simulink library "did"  (R2021b)
settings: Solver=VariableStepAuto  StartTime=0.0  StopTime=10.0  RelTol=1e-3
undefined symbols (not defined in the file or in its folder): ADID_DODRange_pct, ADID_SOCRange_pct, ADID_TempRange_C, DiscIntNeverNeededParam, ENUM_CHRGPLUGSTA_AC, ENUM_CHRGPLUGSTA_DC, ENUM_CHRGPLUGSTA_NONE, ENUM_DRIVETRAIN_AWD, ENUM_DRIVETRAIN_FWD, ENUM_DRIVETRAIN_RWD, ENUM_EXTCHRGSTS_CHARGING, ENUM_OBCV2LSTA_WORKING, ENUM_PWRSTASW_READY, ENUM_VEHICLETYPE_D31HAWD, ENUM_VEHICLETYPE_D31HRWD, HOUR2SEC, HUNDRED, KDID_CPSAVehSpdThres_kph, KDID_DIDModelVersion_raw, KDID_DoDChrgCycle_s, KDID_FiveKmEquivEnergy_Wh, KDID_FlashInitDIDModelVersion_raw, KDID_IPSAVehSpdThres_kph, KDID_PropActiveTripThres_s, KDID_PSARResetThres_sec, KDID_RESSCNTSDODRNGAXIS_enum, KDID_RESSTIMESOCRNGAXIS_enum, KDID_RESSTTEMPRNGAXIS_enum, KDID_WarnUpPropActiveThres_s, KDID_WarnUpVehOperIdleThres_mph, KDID_WarnUpVehOperIdleThres_s, KDID_WarnUpVehOperThres_mph, KDID_WarnUpVehOperThres_s, KPH2MPH, KXX2XX, MINUSONE_FLOAT, ONE_FLOAT, ONE_INT, ONE_INT16, ONE_PERCENT, TRUE, UINT16_MAX, UINT32_MAX, XX2KXX, ZERO_FLOAT, ZERO_INT, ZERO_INT16, ZERO_INT32
libraries: hcu_lib x112, simulink x10, nmm x1
(part 4 of 4)

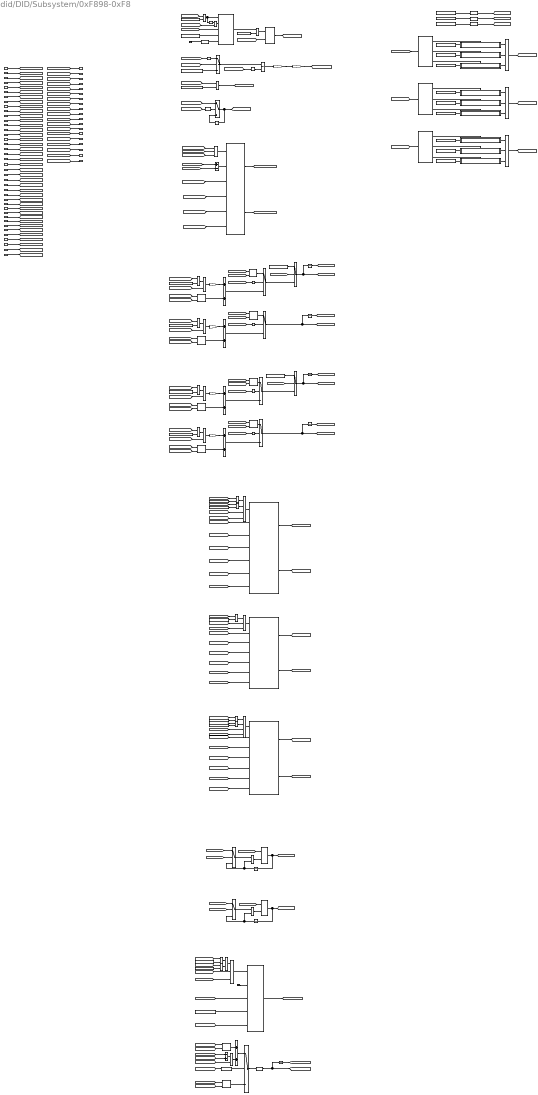
== system did/DID/Subsystem/0xF898-0xF8 ==
  note: 0xF89C: Electric Traction Motor A Total Output Energy
  note: 0xF898, 0xF899: Energy Storage System Depth of Discharge Counter
  note: 0xF89A: Energy Storage System Tracking Tables
  note: 0xF89D: Electric Traction Motor B Total Output Energy
  note: 0xF895: Average Battery Pack Temperature
  note: 0xF894: Minimum and Maximum Pack Temperature
  note: 0xF8A9-E: Energy Storage Accumulated Time at State of Charge
  VDID_HVBattPwr_kW : Inport
  task_time_s : Inport  Port=2
  VINP_CANMsgValidBMS1_flg : Inport  Port=3
  VDID_NoteAResetCondition_flg : Inport  Port=4
  VINP_FlashRESSCNTDODRNGR_cnt : Inport  Port=5
  VINP_FlashRESSCNTDODRNGL_cnt : Inport  Port=6
  VINP_RrMCUDCBusCurr_A : Inport  Port=7
  VINP_RrMCUDCBusVolt_V : Inport  Port=8
  VINP_FlashETMATOER_kWh : Inport  Port=9
  VINP_FlashETMATOEL_kWh : Inport  Port=10
  VINP_CANMsgValidMCUBR1_flg : Inport  Port=11
  VINP_FrMCUDCBusCurr_A : Inport  Port=12
  VINP_FrMCUDCBusVolt_V : Inport  Port=13
  VINP_FlashETMBTOER_kWh : Inport  Port=14
  VINP_FlashETMBTOEL_kWh : Inport  Port=15
  VINP_CANMsgValidMCUBF1_flg : Inport  Port=16
  VPMM_SysPowerMode_enum : Inport  Port=17
  VINP_ChrgPlugSta_enum : Inport  Port=18
  VINP_CANMsgValidBMS6_flg : Inport  Port=19
  VINP_HVBattSOC_pct : Inport  Port=20
  VINP_FlashRESSTIMESOCPSARNGR_s : Inport  Port=21
  VINP_FlashRESSTIMESOCPSARNGL_s : Inport  Port=22
  VINP_ExtChrgSta_enum : Inport  Port=23
  VINP_FlashRESSTIMESOCCHGRNGR_s : Inport  Port=24
  VINP_FlashRESSTIMESOCCHGRNGL_s : Inport  Port=25
  VINP_FlashRESSTIMESOCOFFRNGR_s : Inport  Port=26
  VINP_FlashRESSTIMESOCOFFRNGL_s : Inport  Port=27
  VDID_FlashMAXBATTEMPL_C : Inport  Port=28
  VINP_HVBMTempMax_C : Inport  Port=29
  VINP_CANMsgValidMETER1_flg : Inport  Port=30
  VDID_FlashMINBATTEMPL_C : Inport  Port=31
  VINP_HVBMTempMin_C : Inport  Port=32
  VINP_CANMsgValidBMS4_flg : Inport  Port=33
  VINP_FlashAVGBATTEMPL_sec : Inport  Port=34
  VDID_FlashAVGBATTEMPL_C : Inport  Port=35
  VINP_CellTempAvg_C : Inport  Port=36
  VDID_HVBattPwrDischrg_kW : Inport  Port=37
  VINP_MCUBRRealPwrKwSta_kW : Inport  Port=38
  VINP_MCUBFRealPwrKwSta_kW : Inport  Port=39
  VINP_CANMsgValidBMS3_flg : Inport  Port=40
  AND13 : Logic  Inputs=4  AllPortsSameDT=off  OutDataTypeStr=boolean
  AND3 : Logic  Inputs=3  AllPortsSameDT=off  OutDataTypeStr=boolean
  Abs : Abs
  Add{,1..3} (4 alike) : Sum
  Constant{1,3,7,14,16,51,59,62} (8 alike) : Constant  Value=ZERO_FLOAT
  Constant10 : Constant  Value=KDID_FiveKmEquivEnergy_Wh
  Constant11 : Constant  Value=ADID_DODRange_pct
  Constant116 : Constant  Value=ENUM_CHRGPLUGSTA_NONE
  Constant12 : Constant  Value=zeros(1,7)  OutDataTypeStr=single
  Constant120 : Constant  Value=ENUM_PWRSTASW_READY
  Constant124 : Constant  Value=ENUM_PWRSTASW_READY
  Constant125 : Constant  Value=UINT32_MAX
  Constant13 : Constant  Value=ADID_DODRange_pct
  Constant17 : Constant  Value=KDID_RESSTTEMPRNGAXIS_enum
  Constant18 : Constant  Value=KDID_RESSTIMESOCRNGAXIS_enum
  Constant19 : Constant  Value=KDID_RESSCNTSDODRNGAXIS_enum
  Constant2 : Constant  Value=ADID_SOCRange_pct
  Constant4 : Constant  Value=ADID_TempRange_C
  Constant47 : Constant  Value=ENUM_EXTCHRGSTS_CHARGING
  Constant5 : Constant  Value=zeros(1,5)  OutDataTypeStr=single
  Constant52 : Constant  Value=realmax('single')
  Constant53 : Constant  Value=KDID_DoDChrgCycle_s
  Constant6 : Constant  Value=ADID_TempRange_C
  Constant8 : Constant  Value=zeros(1,7)  OutDataTypeStr=single
  Constant82 : Constant  Value=ENUM_EXTCHRGSTS_CHARGING
  Constant89 : Constant  Value=ENUM_PWRSTASW_READY
  Constant9 : Constant  Value=ADID_SOCRange_pct
  Constant92 : Constant  Value=ENUM_CHRGPLUGSTA_NONE
  Data Type Conversion : DataTypeConversion  OutDataTypeStr=uint8
  Data Type Conversion1 : DataTypeConversion  OutDataTypeStr=single
  Data Type Conversion2 : DataTypeConversion  OutDataTypeStr=uint8
  Data Type Conversion3 : DataTypeConversion  OutDataTypeStr=uint8
  Data Type Conversion4 : DataTypeConversion  OutDataTypeStr=single
  Delay : Delay  DelayLength=1
  Detect Increase : simulink/Logic and Bit Operations/Detect Increase  vinit=0.0  OutDataTypeStr=boolean
  Discrete-Time Integrator : DiscreteIntegrator  ExternalReset=rising  SampleTime=-1  ICPrevOutput=DiscIntNeverNeededParam  ICPrevScaledInput=DiscIntNeverNeededParam
  Divide4 : Product  Inputs=*/
  Equal1 : RelationalOperator  OutDataTypeStr=boolean  RndMeth=Simplest
  Equal{13,27,33,35,54,59} (6 alike) : RelationalOperator  Operator===  OutDataTypeStr=boolean  RndMeth=Simplest
  Equal16 : RelationalOperator  Operator=<  OutDataTypeStr=boolean  RndMeth=Simplest
  Equal17 : RelationalOperator  Operator=>  OutDataTypeStr=boolean  RndMeth=Simplest
  Equal56 : RelationalOperator  Operator=~=  OutDataTypeStr=boolean  RndMeth=Simplest
  Gain{,2..4,10} (5 alike) : Gain  Gain=1/HOUR2SEC
  Gain1 : Gain  Gain=KXX2XX
  Ground : Ground
  Ground1 : Ground
  Initial Value{1..8,11,13,15..16} (12 alike) : hcu_lib/Basic_Blocks/Initial Value
  Logical Operator : Logic  Inputs=3  AllPortsSameDT=off  OutDataTypeStr=boolean
  Logical Operator1 : Logic  Operator=OR  AllPortsSameDT=off  OutDataTypeStr=boolean
  Logical Operator11 : Logic  Inputs=4  AllPortsSameDT=off  OutDataTypeStr=boolean
  Logical Operator8 : Logic  Inputs=3  AllPortsSameDT=off  OutDataTypeStr=boolean
  Max1 : MinMax  Inputs=2
  Max2 : MinMax  Function=max  Inputs=2
  Merge3 : Merge  Inputs=3
  Merge4 : Merge  Inputs=3
  Merge5 : Merge  Inputs=3
  Min{1..3,14} (4 alike) : MinMax  Function=max  Inputs=2
  Minus : Sum  Inputs=+-
  NOT{1..5} (5 alike) : Logic  Operator=NOT  AllPortsSameDT=off  OutDataTypeStr=boolean
  OR : Logic  Operator=OR  AllPortsSameDT=off  OutDataTypeStr=boolean
  Product{1..3,8} (4 alike) : Product
  RangeCnt : hcu_lib/Basic_Blocks/RangeCnt
  RangeTimer : hcu_lib/Basic_Blocks/RangeTimer
  RangeTimer1 : hcu_lib/Basic_Blocks/RangeTimer
  RangeTimer2 : hcu_lib/Basic_Blocks/RangeTimer
  Real_DetectChange4 : hcu_lib/Basic_Blocks/Real_DetectChange
  SR_Latch : hcu_lib/Basic_Blocks/SR_Latch
  Seconds_Counter1 : hcu_lib/Basic_Blocks/Seconds_Counter
  Seconds_Counter11 : hcu_lib/Basic_Blocks/Seconds_Counter
  Subtract7 : Sum
  Subtract8 : Sum  Inputs=-+
  Switch{,1..6,8,14,25} (10 alike) : Switch  Criteria=u2 > Threshold
  Switch Case Action Subsystem10 : Subsystem  TreatAsAtomicUnit=on
  Switch Case Action Subsystem11 : Subsystem  TreatAsAtomicUnit=on
  Switch Case Action Subsystem12 : Subsystem  TreatAsAtomicUnit=on
  Switch Case Action Subsystem13 : Subsystem  TreatAsAtomicUnit=on
  Switch Case Action Subsystem14 : Subsystem  TreatAsAtomicUnit=on
  Switch Case Action Subsystem15 : Subsystem  TreatAsAtomicUnit=on
  Switch Case Action Subsystem16 : Subsystem  TreatAsAtomicUnit=on
  Switch Case Action Subsystem17 : Subsystem  TreatAsAtomicUnit=on
  Switch Case Action Subsystem9 : Subsystem  TreatAsAtomicUnit=on
  Switch Case3 : SwitchCase  CaseConditions={0,1}
  Switch Case4 : SwitchCase  CaseConditions={0,1}
  Switch Case5 : SwitchCase  CaseConditions={0,1}
  Switch54 : Switch  Criteria=u2 ~= 0
      settings: AttributesFormatString=<%<Criteria>>
  Unit Delay{,1..6,27} (8 alike) : UnitDelay  SampleTime=-1  HasFrameUpgradeWarning=on
  VDID_RESSCNTDODRNGR_cnt : Outport
  VDID_RESSCNTDODRNGL_cnt : Outport  Port=2
  VDID_ETMATOER_kWh : Outport  Port=3
  VDID_ETMATOEL_kWh : Outport  Port=4
  VDID_ETMBTOER_kWh : Outport  Port=5
  VDID_ETMBTOEL_kWh : Outport  Port=6
  VDID_RESSTIMESOCPSARNGR_s : Outport  Port=7
  VDID_RESSTIMESOCPSARNGL_s : Outport  Port=8
  VDID_RESSTIMESOCCHGRNGR_s : Outport  Port=9
  VDID_RESSTIMESOCCHGRNGL_s : Outport  Port=10
  VDID_RESSTIMESOCOFFRNGR_s : Outport  Port=11
  VDID_RESSTIMESOCOFFRNGL_s : Outport  Port=12
  VDID_MAXBATTEMPL_C : Outport  Port=13
  VDID_MINBATTEMPL_C : Outport  Port=14
  VDID_AVGBATTEMPL_C : Outport  Port=15
  VDID_RESSTTEMPRNGAXIS_enum : Outport  Port=16
  VDID_RESSTIMESOCRNGAXIS_enum : Outport  Port=17
  VDID_RESSCNTSDODRNGAXIS_enum : Outport  Port=18
  VDID_AVGBATTEMPL_sec : Outport  Port=19
  wires:
  [VINP_FlashRESSCNTDODRNGR_cnt] -> RangeCnt/5
  Constant52/1 -> Seconds_Counter1/4
  [task_time_s] -> Seconds_Counter1/3
  Equal16/1 -> Seconds_Counter1/1, NOT4/1
  [VDID_HVBattPwr_kW] -> Equal16/1
  Data Type Conversion4/1 -> Seconds_Counter1/5
  Ground1/1 -> Data Type Conversion4/1
  RangeCnt/1 -> [VDID_RESSCNTDODRNGR_cnt]
  [VDID_NoteAResetCondition_flg] -> RangeCnt/3
  Seconds_Counter1/1 -> Equal17/1
  Constant53/1 -> Equal17/2
  Constant51/1 -> Equal16/2
  RangeCnt/2 -> [VDID_RESSCNTDODRNGL_cnt]
  [VDID_RESSCNTDODTrigger_flg] -> Logical Operator/1
  [VINP_CANMsgValidBMS1_flg] -> Logical Operator/2
  Equal17/1 -> SR_Latch/1
  SR_Latch/1 -> [VDID_DODMonitorActive_flg]
  [ADID_RESSCNTSDODRNGAXIS_pct] -> RangeCnt/4
  Switch Case3/1 -> Switch Case Action Subsystem9/Action
  Merge3/1 -> [ADID_RESSTTEMPRNGAXIS_C]
  [VDID_RESSCNTSDODRNGAXIS_enum] -> Switch Case5/1
  Switch Case Action Subsystem9/1(ADID_RESSTTEMPRNGAXIS_C) -> Merge3/1
  Constant6/1 -> Switch Case Action Subsystem11/1(ADID_TempRange_C)
  Switch Case Action Subsystem14/1(ADID_RESSTIMESOCRNGAXIS_pct) -> Merge4/3
  Constant4/1 -> Switch Case Action Subsystem10/1(ADID_TempRange_C)
  Switch Case Action Subsystem11/1(ADID_RESSTTEMPRNGAXIS_C) -> Merge3/3
  Merge4/1 -> [ADID_RESSTIMESOCRNGAXIS_pct]
  Switch Case Action Subsystem13/1(ADID_RESSTIMESOCRNGAXIS_pct) -> Merge4/2
  Constant5/1 -> Switch Case Action Subsystem9/1(ADID_TempRange_C)
  Switch Case4/3 -> Switch Case Action Subsystem14/Action
  Switch Case Action Subsystem12/1(ADID_RESSTIMESOCRNGAXIS_pct) -> Merge4/1
  Constant11/1 -> Switch Case Action Subsystem16/1(ADID_DODRange_pct)
  Switch Case4/2 -> Switch Case Action Subsystem13/Action
  Switch Case Action Subsystem10/1(ADID_RESSTTEMPRNGAXIS_C) -> Merge3/2
  Switch Case3/2 -> Switch Case Action Subsystem10/Action
  Switch Case4/1 -> Switch Case Action Subsystem12/Action
  Switch Case5/2 -> Switch Case Action Subsystem16/Action
  Switch Case3/3 -> Switch Case Action Subsystem11/Action
  Constant12/1 -> Switch Case Action Subsystem15/1(ADID_DODRange_pct)
  Switch Case Action Subsystem15/1(ADID_RESSCNTSDODRNGAXIS_pct) -> Merge5/1
  Switch Case5/1 -> Switch Case Action Subsystem15/Action
  Merge5/1 -> [ADID_RESSCNTSDODRNGAXIS_pct]
  Constant2/1 -> Switch Case Action Subsystem13/1(ADID_SOCRange_pct)
  Switch Case5/3 -> Switch Case Action Subsystem17/Action
  Constant9/1 -> Switch Case Action Subsystem14/1(ADID_SOCRange_pct)
  Constant13/1 -> Switch Case Action Subsystem17/1(ADID_DODRange_pct)
  Switch Case Action Subsystem16/1(ADID_RESSCNTSDODRNGAXIS_pct) -> Merge5/2
  Constant8/1 -> Switch Case Action Subsystem12/1(ADID_SOCRange_pct)
  Switch Case Action Subsystem17/1(ADID_RESSCNTSDODRNGAXIS_pct) -> Merge5/3
  Initial Value13/1 -> Add/2
  [VDID_NoteAResetCondition_flg] -> Switch14/2
  Switch25/1 -> Switch14/3
  Constant62/1 -> Switch14/1
  NOT1/1 -> Switch25/2
  Add/1 -> Switch25/3
  Switch14/1 -> Unit Delay/1, [VDID_ETMATOER_kWh]
  Unit Delay/1 -> [VDID_DelayETMATOER_kWh]
  [VDID_DelayETMATOER_kWh] -> Initial Value13/2
  [VINP_FlashETMATOER_kWh] -> Initial Value13/1
  Unit Delay1/1 -> [VDID_DelayETMATOEL_kWh]
  [VDID_DelayETMATOEL_kWh] -> Initial Value1/2
  Add1/1 -> Switch2/3
  NOT2/1 -> Switch2/2
  Switch2/1 -> Unit Delay1/1, [VDID_ETMATOEL_kWh]
  [VINP_FlashETMATOEL_kWh] -> Initial Value1/1
  Initial Value1/1 -> Add1/2
  Add2/1 -> Switch4/3
  [VINP_FlashETMBTOER_kWh] -> Initial Value3/1
  Initial Value3/1 -> Add2/2
  Switch3/1 -> Unit Delay3/1, [VDID_ETMBTOEL_kWh]
  Constant16/1 -> Switch1/1
  [VINP_FlashETMBTOEL_kWh] -> Initial Value2/1
  Initial Value2/1 -> Add3/2
  NOT3/1 -> Switch4/2
  Switch1/1 -> Unit Delay2/1, [VDID_ETMBTOER_kWh]
  NOT5/1 -> Switch3/2
  Add3/1 -> Switch3/3
  [VDID_DelayETMBTOEL_kWh] -> Initial Value2/2
  Switch4/1 -> Switch1/3
  Unit Delay2/1 -> [VDID_DelayETMBTOER_kWh]
  [VDID_DelayETMBTOER_kWh] -> Initial Value3/2
  Unit Delay3/1 -> [VDID_DelayETMBTOEL_kWh]
  [VDID_NoteAResetCondition_flg] -> Switch1/2
  [VINP_FlashRESSCNTDODRNGL_cnt] -> RangeCnt/6
  VINP_FlashRESSCNTDODRNGR_cnt/1 -> [VINP_FlashRESSCNTDODRNGR_cnt]
  VINP_RrMCUDCBusCurr_A/1 -> [VINP_RrMCUDCBusCurr_A]
  VINP_FlashETMBTOEL_kWh/1 -> [VINP_FlashETMBTOEL_kWh]
  VINP_FrMCUDCBusCurr_A/1 -> [VINP_FrMCUDCBusCurr_A]
  VINP_ChrgPlugSta_enum/1 -> [VINP_ChrgPlugSta_enum]
  VDID_NoteAResetCondition_flg/1 -> [VDID_NoteAResetCondition_flg]
  VINP_CANMsgValidMCUBR1_flg/1 -> [VINP_CANMsgValidMCUBR1_flg]
  VINP_FlashRESSCNTDODRNGL_cnt/1 -> [VINP_FlashRESSCNTDODRNGL_cnt]
  VINP_CANMsgValidMCUBF1_flg/1 -> [VINP_CANMsgValidMCUBF1_flg]
  VINP_CANMsgValidBMS1_flg/1 -> [VINP_CANMsgValidBMS1_flg]
  VPMM_SysPowerMode_enum/1 -> [VPMM_SysPowerMode_enum]
  VDID_HVBattPwr_kW/1 -> [VDID_HVBattPwr_kW]
  VINP_FlashETMATOER_kWh/1 -> [VINP_FlashETMATOER_kWh]
  [VDID_RESSCNTDODRNGL_cnt] -> VDID_RESSCNTDODRNGL_cnt/1
  VINP_FlashRESSTIMESOCCHGRNGL_s/1 -> [VINP_FlashRESSTIMESOCCHGRNGL_s]
  task_time_s/1 -> [task_time_s]
  [VDID_ETMATOER_kWh] -> VDID_ETMATOER_kWh/1
  VINP_RrMCUDCBusVolt_V/1 -> [VINP_RrMCUDCBusVolt_V]
  VINP_CANMsgValidBMS6_flg/1 -> [VINP_CANMsgValidBMS6_flg]
  VINP_FlashETMBTOER_kWh/1 -> [VINP_FlashETMBTOER_kWh]
  VINP_FlashRESSTIMESOCOFFRNGR_s/1 -> [VINP_FlashRESSTIMESOCOFFRNGR_s]
  VINP_FlashETMATOEL_kWh/1 -> [VINP_FlashETMATOEL_kWh]
  VINP_FlashRESSTIMESOCOFFRNGL_s/1 -> [VINP_FlashRESSTIMESOCOFFRNGL_s]
  [VDID_ETMATOEL_kWh] -> VDID_ETMATOEL_kWh/1
  VINP_ExtChrgSta_enum/1 -> [VINP_ExtChrgSta_enum]
  [VDID_RESSTIMESOCOFFRNGR_s] -> VDID_RESSTIMESOCOFFRNGR_s/1
  VINP_HVBattSOC_pct/1 -> [VINP_HVBattSOC_pct]
  VINP_FlashRESSTIMESOCPSARNGR_s/1 -> [VINP_FlashRESSTIMESOCPSARNGR_s]
  [VDID_RESSTIMESOCPSARNGL_s] -> VDID_RESSTIMESOCPSARNGL_s/1
  VINP_FlashRESSTIMESOCPSARNGL_s/1 -> [VINP_FlashRESSTIMESOCPSARNGL_s]
  [VDID_RESSTIMESOCCHGRNGR_s] -> VDID_RESSTIMESOCCHGRNGR_s/1
  [VDID_ETMBTOER_kWh] -> VDID_ETMBTOER_kWh/1
  [VDID_RESSTIMESOCCHGRNGL_s] -> VDID_RESSTIMESOCCHGRNGL_s/1
  VINP_FlashRESSTIMESOCCHGRNGR_s/1 -> [VINP_FlashRESSTIMESOCCHGRNGR_s]
  [VDID_RESSCNTDODRNGR_cnt] -> VDID_RESSCNTDODRNGR_cnt/1
  [VDID_ETMBTOEL_kWh] -> VDID_ETMBTOEL_kWh/1
  VINP_FrMCUDCBusVolt_V/1 -> [VINP_FrMCUDCBusVolt_V]
  [VDID_RESSTIMESOCOFFRNGL_s] -> VDID_RESSTIMESOCOFFRNGL_s/1
  [VDID_RESSTIMESOCPSARNGR_s] -> VDID_RESSTIMESOCPSARNGR_s/1
  [VINP_FlashAVGBATTEMPL_sec] -> Seconds_Counter11/5
  RangeTimer/2 -> [VDID_RESSTIMESOCPSARNGL_s]
  [VINP_FlashRESSTIMESOCOFFRNGL_s] -> RangeTimer2/7
  Equal54/1 -> AND13/2
  [VINP_CANMsgValidBMS6_flg] -> AND3/3
  [VINP_CANMsgValidBMS4_flg] -> AND3/2
  Data Type Conversion1/1 -> [VDID_AVGBATTEMPL_C], Unit Delay27/1
  [VINP_ChrgPlugSta_enum] -> Equal54/1
  [VINP_ExtChrgSta_enum] -> Equal27/1
  [VDID_NoteAResetCondition_flg] -> RangeTimer1/4
  [VDID_FlashAVGBATTEMPL_C] -> Initial Value15/1
  [VINP_HVBattSOC_pct] -> RangeTimer2/2
  [VDID_AVGBATTEMPL_sec] -> Real_DetectChange4/1
  [VINP_ExtChrgSta_enum] -> Equal13/1
  Seconds_Counter11/1 -> [VDID_AVGBATTEMPL_sec]
  [VDID_FlashAVGBATTEMPL_C] -> Initial Value16/1
  Constant47/1 -> Equal13/2
  Initial Value15/1 -> Subtract7/1
  [VDID_AVGBATTEMPL_sec] -> Divide4/2
  AND3/1 -> Seconds_Counter11/1
  Constant125/1 -> Seconds_Counter11/4
  [ADID_RESSTIMESOCRNGAXIS_pct] -> RangeTimer/5
  Constant120/1 -> Equal56/2
  Equal56/1 -> AND13/1
  [task_time_s] -> Seconds_Counter11/3
  [VINP_CANMsgValidBMS6_flg] -> Logical Operator8/2
  [VDID_DelayAVGBATTEMPL_C] -> Initial Value16/2
  Initial Value16/1 -> Switch54/3
  [ADID_RESSTIMESOCRNGAXIS_pct] -> RangeTimer1/5
  Logical Operator8/1 -> RangeTimer1/1
  RangeTimer2/2 -> [VDID_RESSTIMESOCOFFRNGL_s]
  [VINP_FlashRESSTIMESOCPSARNGL_s] -> RangeTimer/7
  [VINP_FlashRESSTIMESOCCHGRNGR_s] -> RangeTimer1/6
  [task_time_s] -> RangeTimer1/3
  [VDID_NoteAResetCondition_flg] -> RangeTimer/4
  [VINP_HVBattSOC_pct] -> RangeTimer/2
  RangeTimer/1 -> [VDID_RESSTIMESOCPSARNGR_s]
  [VINP_CANMsgValidBMS4_flg] -> Switch5/2
  Switch54/1 -> Data Type Conversion1/1
  RangeTimer2/1 -> [VDID_RESSTIMESOCOFFRNGR_s]
  [VINP_FlashRESSTIMESOCCHGRNGL_s] -> RangeTimer1/7
  [ADID_RESSTIMESOCRNGAXIS_pct] -> RangeTimer2/5
  [VDID_NoteAResetCondition_flg] -> RangeTimer2/4
  [VINP_CANMsgValidBMS6_flg] -> Logical Operator11/3
  Subtract7/1 -> Switch54/1
  Unit Delay27/1 -> [VDID_DelayAVGBATTEMPL_C]
  Divide4/1 -> Subtract7/2
  Constant124/1 -> Equal59/2
  [VINP_FlashRESSTIMESOCPSARNGR_s] -> RangeTimer/6
  AND13/1 -> RangeTimer2/1
  [VDID_DelayAVGBATTEMPL_C] -> Subtract8/1
  Equal27/1 -> Logical Operator8/1
  RangeTimer1/1 -> [VDID_RESSTIMESOCCHGRNGR_s]
  [VINP_ChrgPlugSta_enum] -> Equal35/1
  [VINP_CellTempAvg_C] -> Subtract8/2
  Real_DetectChange4/1 -> Switch54/2
  Unit Delay5/1 -> Switch5/3, Max1/2
  Constant82/1 -> Equal27/2
  Constant92/1 -> Equal35/2
  [VDID_DelayAVGBATTEMPL_C] -> Initial Value15/2
  [VINP_HVBattSOC_pct] -> RangeTimer1/2
  [VINP_HVBMTempMin_C] -> Switch5/1
  Subtract8/1 -> Divide4/1
  [VPMM_SysPowerMode_enum] -> Equal33/1
  RangeTimer1/2 -> [VDID_RESSTIMESOCCHGRNGL_s]
  [VINP_HVBMTempMax_C] -> Switch6/1
  [task_time_s] -> RangeTimer2/3
  [VINP_CANMsgValidBMS6_flg] -> AND13/3
  Equal35/1 -> Logical Operator11/2
  [VPMM_SysPowerMode_enum] -> Equal56/1
  Logical Operator11/1 -> RangeTimer/1
  [VPMM_SysPowerMode_enum] -> Equal59/1
  [VINP_FlashRESSTIMESOCOFFRNGR_s] -> RangeTimer2/6
  [task_time_s] -> RangeTimer/3
  Constant89/1 -> Equal33/2
  Equal33/1 -> Logical Operator11/1
  Constant116/1 -> Equal54/2
  VDID_FlashMAXBATTEMPL_C/1 -> [VDID_FlashMAXBATTEMPL_C]
  VINP_CANMsgValidBMS4_flg/1 -> [VINP_CANMsgValidBMS4_flg]
  VDID_FlashMINBATTEMPL_C/1 -> [VDID_FlashMINBATTEMPL_C]
  VINP_FlashAVGBATTEMPL_sec/1 -> [VINP_FlashAVGBATTEMPL_sec]
  VINP_CANMsgValidMETER1_flg/1 -> [VINP_CANMsgValidMETER1_flg]
  VDID_FlashAVGBATTEMPL_C/1 -> [VDID_FlashAVGBATTEMPL_C]
  VINP_HVBMTempMax_C/1 -> [VINP_HVBMTempMax_C]
  VINP_CellTempAvg_C/1 -> [VINP_CellTempAvg_C]
  VINP_HVBMTempMin_C/1 -> [VINP_HVBMTempMin_C]
  [VDID_AVGBATTEMPL_C] -> VDID_AVGBATTEMPL_C/1
  [VDID_MINBATTEMPL_C] -> VDID_MINBATTEMPL_C/1
  [VDID_MAXBATTEMPL_C] -> VDID_MAXBATTEMPL_C/1
  [VDID_RESSTTEMPRNGAXIS_enum] -> Switch Case3/1
  [VDID_RESSTIMESOCRNGAXIS_enum] -> Switch Case4/1
  VDID_HVBattPwrDischrg_kW/1 -> [VDID_HVBattPwrDischrg_kW]
  [VDID_DODMonitorActive_flg] -> Switch/2
  Constant7/1 -> Switch/3
  [VDID_HVBattPwrDischrg_kW] -> Abs/1
  Discrete-Time Integrator/1 -> Gain1/1
  Switch/1 -> Discrete-Time Integrator/1
  Gain1/1 -> Gain/1
  Gain/1 -> [VDID_HVBatteEnergyDischrg_Wh]
  [VDID_HVBatteEnergyDischrg_Wh] -> Equal1/1
  Constant10/1 -> Equal1/2
  Equal1/1 -> [VDID_RESSCNTDODTrigger_flg]
  [VDID_RESSCNTDODTrigger_flg] -> SR_Latch/2
  OR/1 -> Seconds_Counter1/2
  NOT4/1 -> OR/1
  [VDID_RESSCNTDODTrigger_flg] -> OR/2
  [VINP_HVBattSOC_pct] -> Switch8/1
  Unit Delay6/1 -> Switch8/3
  Detect Increase/1 -> Switch8/2
  [VDID_DODMonitorActive_flg] -> Detect Increase/1
  Switch8/1 -> [VDID_SOCStart_pct], Unit Delay6/1
  Logical Operator/1 -> RangeCnt/1
  Minus/1 -> RangeCnt/2
  [VDID_SOCStart_pct] -> Minus/2
  [VINP_HVBattSOC_pct] -> Minus/1
  Ground/1 -> Seconds_Counter11/2
  VINP_MCUBRRealPwrKwSta_kW/1 -> [VINP_MCUBRRealPwrKwSta_kW]
  Constant59/1 -> Min14/2
  [VINP_MCUBFRealPwrKwSta_kW] -> Min14/1
  [task_time_s] -> Product8/2
  Min14/1 -> Product8/1
  Product8/1 -> Gain10/1
  Gain10/1 -> Add/1
  Gain2/1 -> Add1/1
  [task_time_s] -> Product1/2
  Min1/1 -> Product1/1
  Constant1/1 -> Min1/2
  Product1/1 -> Gain2/1
  [VDID_RESSTTEMPRNGAXIS_enum] -> VDID_RESSTTEMPRNGAXIS_enum/1
  [VDID_RESSTIMESOCRNGAXIS_enum] -> VDID_RESSTIMESOCRNGAXIS_enum/1
  [VDID_RESSCNTSDODRNGAXIS_enum] -> VDID_RESSCNTSDODRNGAXIS_enum/1
  [VINP_MCUBRRealPwrKwSta_kW] -> Min2/1
  Min2/1 -> Product2/1
  Gain3/1 -> Add2/1
  [task_time_s] -> Product2/2
  Product2/1 -> Gain3/1
  Constant3/1 -> Min2/2
  Constant14/1 -> Min3/2
  Product3/1 -> Gain4/1
  [task_time_s] -> Product3/2
  [VINP_MCUBRRealPwrKwSta_kW] -> Min3/1
  Min3/1 -> Product3/1
  Gain4/1 -> Add3/1
  [VINP_MCUBFRealPwrKwSta_kW] -> Min1/1
  VINP_MCUBFRealPwrKwSta_kW/1 -> [VINP_MCUBFRealPwrKwSta_kW]
  [VINP_CANMsgValidBMS3_flg] -> Logical Operator/3
  VINP_CANMsgValidBMS3_flg/1 -> [VINP_CANMsgValidBMS3_flg]
  [VINP_CANMsgValidBMS3_flg] -> Logical Operator11/4
  [VINP_CANMsgValidBMS3_flg] -> Logical Operator8/3
  [VINP_CANMsgValidBMS3_flg] -> AND13/4
  Constant17/1 -> Data Type Conversion2/1
  Data Type Conversion2/1 -> [VDID_RESSTTEMPRNGAXIS_enum]
  Constant19/1 -> Data Type Conversion3/1
  Data Type Conversion3/1 -> [VDID_RESSCNTSDODRNGAXIS_enum]
  Constant18/1 -> Data Type Conversion/1
  Data Type Conversion/1 -> [VDID_RESSTIMESOCRNGAXIS_enum]
  [VDID_AVGBATTEMPL_sec] -> VDID_AVGBATTEMPL_sec/1
  [VINP_FlashETMATOER_kWh] -> Initial Value5/1
  [VDID_DelayETMATOER_kWh] -> Initial Value5/2
  Initial Value5/1 -> Switch25/1
  [VDID_DelayETMATOEL_kWh] -> Initial Value6/2
  [VINP_FlashETMATOEL_kWh] -> Initial Value6/1
  Initial Value6/1 -> Switch2/1
  [VINP_FlashETMBTOER_kWh] -> Initial Value7/1
  [VDID_DelayETMBTOER_kWh] -> Initial Value7/2
  Initial Value7/1 -> Switch4/1
  [VINP_FlashETMBTOEL_kWh] -> Initial Value8/1
  [VDID_DelayETMBTOEL_kWh] -> Initial Value8/2
  Initial Value8/1 -> Switch3/1
  Switch5/1 -> Max1/1
  Max1/1 -> Initial Value11/2
  [VDID_FlashMINBATTEMPL_C] -> Initial Value11/1
  Initial Value11/1 -> Unit Delay5/1, [VDID_MINBATTEMPL_C]
  Initial Value4/1 -> [VDID_MAXBATTEMPL_C], Unit Delay4/1
  Max2/1 -> Initial Value4/2
  Switch6/1 -> Max2/1
  Unit Delay4/1 -> Max2/2, Switch6/3
  [VDID_FlashMAXBATTEMPL_C] -> Initial Value4/1
  [VINP_CANMsgValidBMS4_flg] -> Switch6/2
  Equal59/1 -> Logical Operator1/1
  Equal13/1 -> Logical Operator1/2
  Logical Operator1/1 -> AND3/1
  Abs/1 -> Switch/1
  [VDID_RESSCNTDODTrigger_flg] -> Delay/1
  Delay/1 -> Discrete-Time Integrator/2
  [VINP_CANMsgValidMCUBR1_flg] -> NOT3/1
  [VINP_CANMsgValidMCUBR1_flg] -> NOT5/1
  [VINP_CANMsgValidMCUBF1_flg] -> NOT2/1
  [VINP_CANMsgValidMCUBF1_flg] -> NOT1/1

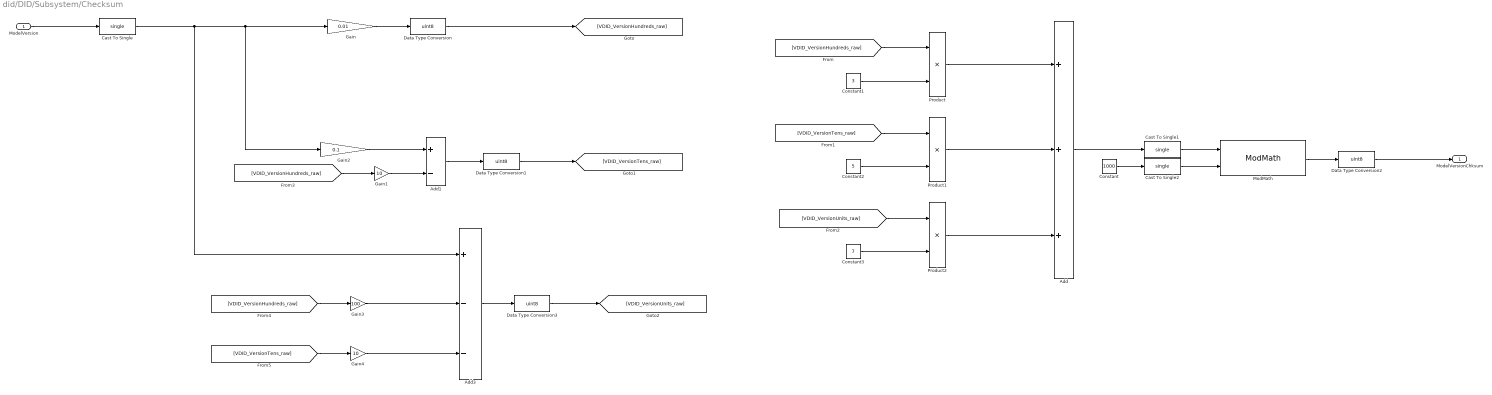
== system did/DID/Subsystem/Checksum ==
  ModelVersion : Inport
  Add : Sum  Inputs=+++
  Add1 : Sum  Inputs=+-
  Add3 : Sum  Inputs=+--
  Cast To Single : DataTypeConversion  OutDataTypeStr=single
  Cast To Single1 : DataTypeConversion  OutDataTypeStr=single
  Cast To Single2 : DataTypeConversion  OutDataTypeStr=single
  Constant : Constant  Value=1000
  Constant1 : Constant  Value=3
  Constant2 : Constant  Value=5
  Constant3 : Constant  Value=7
  Data Type Conversion{,1..3} (4 alike) : DataTypeConversion  OutDataTypeStr=uint8
  Gain : Gain  Gain=0.01
  Gain1 : Gain  Gain=10
  Gain2 : Gain  Gain=0.1
  Gain3 : Gain  Gain=100
  Gain4 : Gain  Gain=10
  ModMath : hcu_lib/Basic_Blocks/ModMath
  Product : Product
  Product1 : Product
  Product2 : Product
  ModelVersionChksum : Outport
  wires:
  Cast To Single1/1 -> ModMath/1
  Cast To Single2/1 -> ModMath/2
  [VDID_VersionHundreds_raw] -> Gain3/1
  Gain/1 -> Data Type Conversion/1
  Add1/1 -> Data Type Conversion1/1
  Product1/1 -> Add/2
  Gain2/1 -> Add1/1
  Add3/1 -> Data Type Conversion3/1
  Data Type Conversion2/1 -> ModelVersionChksum/1
  Data Type Conversion/1 -> [VDID_VersionHundreds_raw]
  [VDID_VersionTens_raw] -> Product1/1
  [VDID_VersionUnits_raw] -> Product2/1
  Constant1/1 -> Product/2
  Gain1/1 -> Add1/2
  Data Type Conversion3/1 -> [VDID_VersionUnits_raw]
  Add/1 -> Cast To Single1/1
  [VDID_VersionHundreds_raw] -> Gain1/1
  ModelVersion/1 -> Cast To Single/1
  Constant/1 -> Cast To Single2/1
  Product/1 -> Add/1
  ModMath/1 -> Data Type Conversion2/1
  Constant3/1 -> Product2/2
  Gain3/1 -> Add3/2
  Cast To Single/1 -> Gain/1, Gain2/1, Add3/1
  Data Type Conversion1/1 -> [VDID_VersionTens_raw]
  Constant2/1 -> Product1/2
  [VDID_VersionTens_raw] -> Gain4/1
  Gain4/1 -> Add3/3
  [VDID_VersionHundreds_raw] -> Product/1
  Product2/1 -> Add/3

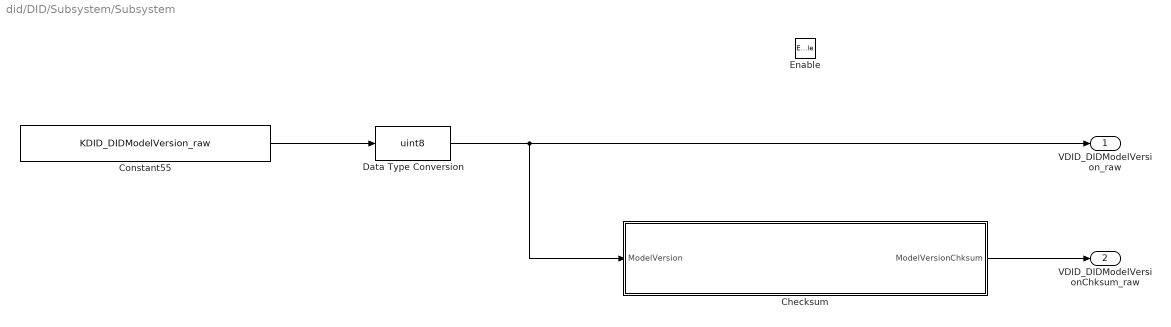
== system did/DID/Subsystem/Subsystem ==
  Enable : EnablePort
  Checksum : Subsystem
  Constant55 : Constant  Value=KDID_DIDModelVersion_raw
  Data Type Conversion : DataTypeConversion  OutDataTypeStr=uint8
  VDID_DIDModelVersion_raw : Outport
  VDID_DIDModelVersionChksum_raw : Outport  Port=2
  wires:
  Checksum/1(ModelVersionChksum) -> VDID_DIDModelVersionChksum_raw/1
  Constant55/1 -> Data Type Conversion/1
  Data Type Conversion/1 -> Checksum/1(ModelVersion), VDID_DIDModelVersion_raw/1

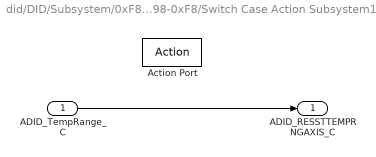
== system did/DID/Subsystem/0xF898-0xF8/Switch Case Action Subsystem10 ==
  ADID_TempRange_C : Inport
  Action Port : ActionPort  ActionPortLabel=case [ 1 ]:
  ADID_RESSTTEMPRNGAXIS_C : Outport
  wires:
  ADID_TempRange_C/1 -> ADID_RESSTTEMPRNGAXIS_C/1

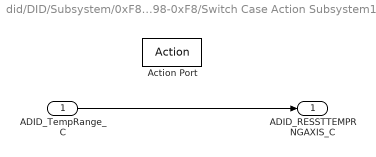
== system did/DID/Subsystem/0xF898-0xF8/Switch Case Action Subsystem11 ==
  ADID_TempRange_C : Inport
  Action Port : ActionPort  ActionPortLabel=default:
  ADID_RESSTTEMPRNGAXIS_C : Outport
  wires:
  ADID_TempRange_C/1 -> ADID_RESSTTEMPRNGAXIS_C/1

== system did/DID/Subsystem/0xF898-0xF8/Switch Case Action Subsystem12 ==
  ADID_SOCRange_pct : Inport
  Action Port : ActionPort  ActionPortLabel=case [ 0 ]:
  ADID_RESSTIMESOCRNGAXIS_pct : Outport
  wires:
  ADID_SOCRange_pct/1 -> ADID_RESSTIMESOCRNGAXIS_pct/1

== system did/DID/Subsystem/0xF898-0xF8/Switch Case Action Subsystem13 ==
  ADID_SOCRange_pct : Inport
  Action Port : ActionPort  ActionPortLabel=case [ 1 ]:
  ADID_RESSTIMESOCRNGAXIS_pct : Outport
  wires:
  ADID_SOCRange_pct/1 -> ADID_RESSTIMESOCRNGAXIS_pct/1

== system did/DID/Subsystem/0xF898-0xF8/Switch Case Action Subsystem14 ==
  ADID_SOCRange_pct : Inport
  Action Port : ActionPort  ActionPortLabel=default:
  ADID_RESSTIMESOCRNGAXIS_pct : Outport
  wires:
  ADID_SOCRange_pct/1 -> ADID_RESSTIMESOCRNGAXIS_pct/1

== system did/DID/Subsystem/0xF898-0xF8/Switch Case Action Subsystem15 ==
  ADID_DODRange_pct : Inport
  Action Port : ActionPort  ActionPortLabel=case [ 0 ]:
  ADID_RESSCNTSDODRNGAXIS_pct : Outport
  wires:
  ADID_DODRange_pct/1 -> ADID_RESSCNTSDODRNGAXIS_pct/1

== system did/DID/Subsystem/0xF898-0xF8/Switch Case Action Subsystem16 ==
  ADID_DODRange_pct : Inport
  Action Port : ActionPort  ActionPortLabel=case [ 1 ]:
  ADID_RESSCNTSDODRNGAXIS_pct : Outport
  wires:
  ADID_DODRange_pct/1 -> ADID_RESSCNTSDODRNGAXIS_pct/1

== system did/DID/Subsystem/0xF898-0xF8/Switch Case Action Subsystem17 ==
  ADID_DODRange_pct : Inport
  Action Port : ActionPort  ActionPortLabel=default:
  ADID_RESSCNTSDODRNGAXIS_pct : Outport
  wires:
  ADID_DODRange_pct/1 -> ADID_RESSCNTSDODRNGAXIS_pct/1

== system did/DID/Subsystem/0xF898-0xF8/Switch Case Action Subsystem9 ==
  ADID_TempRange_C : Inport
  Action Port : ActionPort  ActionPortLabel=case [ 0 ]:
  ADID_RESSTTEMPRNGAXIS_C : Outport
  wires:
  ADID_TempRange_C/1 -> ADID_RESSTTEMPRNGAXIS_C/1

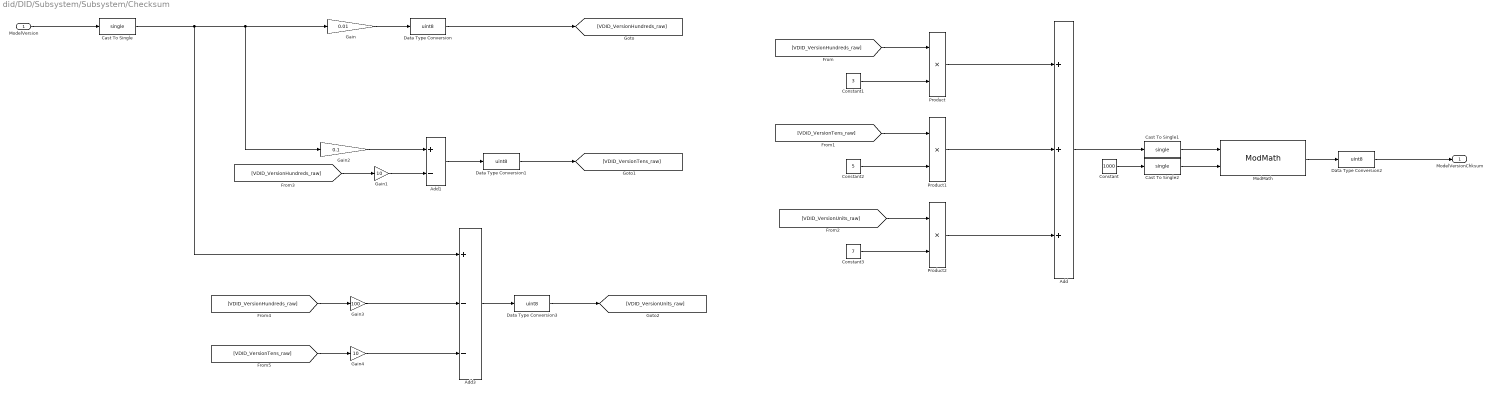
== system did/DID/Subsystem/Subsystem/Checksum ==
  ModelVersion : Inport
  Add : Sum  Inputs=+++
  Add1 : Sum  Inputs=+-
  Add3 : Sum  Inputs=+--
  Cast To Single : DataTypeConversion  OutDataTypeStr=single
  Cast To Single1 : DataTypeConversion  OutDataTypeStr=single
  Cast To Single2 : DataTypeConversion  OutDataTypeStr=single
  Constant : Constant  Value=1000
  Constant1 : Constant  Value=3
  Constant2 : Constant  Value=5
  Constant3 : Constant  Value=7
  Data Type Conversion{,1..3} (4 alike) : DataTypeConversion  OutDataTypeStr=uint8
  Gain : Gain  Gain=0.01
  Gain1 : Gain  Gain=10
  Gain2 : Gain  Gain=0.1
  Gain3 : Gain  Gain=100
  Gain4 : Gain  Gain=10
  ModMath : hcu_lib/Basic_Blocks/ModMath
  Product : Product
  Product1 : Product
  Product2 : Product
  ModelVersionChksum : Outport
  wires:
  Product2/1 -> Add/3
  [VDID_VersionHundreds_raw] -> Product/1
  Gain4/1 -> Add3/3
  [VDID_VersionTens_raw] -> Gain4/1
  Constant2/1 -> Product1/2
  Data Type Conversion1/1 -> [VDID_VersionTens_raw]
  Cast To Single/1 -> Add3/1, Gain2/1, Gain/1
  Gain3/1 -> Add3/2
  Constant3/1 -> Product2/2
  ModMath/1 -> Data Type Conversion2/1
  Product/1 -> Add/1
  Constant/1 -> Cast To Single2/1
  ModelVersion/1 -> Cast To Single/1
  [VDID_VersionHundreds_raw] -> Gain1/1
  Add/1 -> Cast To Single1/1
  Data Type Conversion3/1 -> [VDID_VersionUnits_raw]
  Gain1/1 -> Add1/2
  Constant1/1 -> Product/2
  [VDID_VersionUnits_raw] -> Product2/1
  [VDID_VersionTens_raw] -> Product1/1
  Data Type Conversion/1 -> [VDID_VersionHundreds_raw]
  Data Type Conversion2/1 -> ModelVersionChksum/1
  Add3/1 -> Data Type Conversion3/1
  Gain2/1 -> Add1/1
  Product1/1 -> Add/2
  Add1/1 -> Data Type Conversion1/1
  Gain/1 -> Data Type Conversion/1
  [VDID_VersionHundreds_raw] -> Gain3/1
  Cast To Single2/1 -> ModMath/2
  Cast To Single1/1 -> ModMath/1

== stateflow chart did/DID/Subsystem/Scheduler1 ==
  state trigger_1sec
    (default) -> (junction 63) : {
        | counter = 0;
        | }
    trigger_1sec -> (junction 63)
    (junction 63) -> (junction 41) [order 1] : [trigger]
    (junction 63) -> (junction 68) [order 2] : {
        | trig_1sec = 0;
        | }
    (junction 41) -> (junction 1) : {
        | counter++;
        | }
    (junction 1) -> (junction 8) [order 1] : [counter%%uint32(1/task_time_s) == 0]  /* 1sec trigger */
    (junction 1) -> (junction 5) [order 2] : {
        | trig_1sec = 0;
        | }
    (junction 8) -> (junction 9) : {
        | trig_1sec = 1;
        | counter = 0;
        | }
  data: counter local uint32 size=1; task_time_s input; trigger input; trig_1sec output boolean

== stateflow chart did/DID/Subsystem/Scheduler ==
  state trigger_1sec
    (default) -> (junction 63) : {
        | counter = 0;
        | }
    trigger_1sec -> (junction 63)
    (junction 63) -> (junction 41) [order 1] : [trigger]
    (junction 63) -> (junction 68) [order 2] : {
        | trig_1sec = 0;
        | }
    (junction 41) -> (junction 1) : {
        | counter++;
        | }
    (junction 1) -> (junction 8) [order 1] : [counter%%uint32(1/task_time_s) == 0]  /* 1sec trigger */
    (junction 1) -> (junction 5) [order 2] : {
        | trig_1sec = 0;
        | }
    (junction 8) -> (junction 9) : {
        | trig_1sec = 1;
        | counter = 0;
        | }
  data: counter local uint32 size=1; task_time_s input; trigger input; trig_1sec output boolean
